simulink model "PendulumCart_Block"  (R2020a)
settings: Solver=ode45  StartTime=0.0  StopTime=12  RelTol=1e-3  EnableMultiTasking=on
values from neighbouring files (symbols this model uses):
  calGain = 1/dcgain(cltf)    [TP.m]
  g = 9.81    [TP.m]
  K = acker(A,B,phi)    [TP.m]
  l = 1    [TP.m]
  m = 0.5    [TP.m]
  M = 2    [TP.m]
  theta_0 = 0    [TP.m]
  theta_dot_0 = 0    [TP.m]
  x_0 = 0    [TP.m]
  x_dot_0 = 0    [TP.m]
settings Model: Creator=rodrigue  LastModifiedBy=m214134
settings DataIOCC: LimitDataPoints=on  SaveFormat=Array  ReturnWorkspaceOutputs=off
settings OptimizationCC: LifeSpan=inf
settings DebuggingCC: UnderspecifiedInitializationDetection=Classic  MergeDetectMultiDrivingBlocksExec=none  SolverPrmCheckMsg=warning  StateNameClashWarn=warning  SFUnexpectedBacktrackingDiag=warning  SFNoUnconditionalDefaultTransitionDiag=warning  SFExecutionAtInitializationDiag=none  ArithmeticOperatorsInVariantConditions=warning
settings HardwareCC: ProdBitPerPointer=32  ProdBitPerSizeT=32  ProdBitPerPtrDiffT=32  ProdLargestAtomicFloat=None  ProdIntDivRoundTo=Undefined  ProdEndianess=Unspecified  ProdWordSize=32  ProdHWDeviceType=32-bit Generic
settings ModelReferenceCC: PropagateSignalLabelsOutOfModel=off
settings SFSimCC: SimUseLocalCustomCode=off  CustomCodeUndefinedFunction=UseInterfaceOnly
settings RTWCC: RTWUseLocalCustomCode=off
settings CodeAppCC: StateflowObjectComments=on
settings GRTTargetCC: TargetLangStandard=C89/C90 (ANSI)
settings ConfigComp: CovMetricSettings=dw  CovHtmlReporting=on  CovSaveCumulativeToWorkspaceVar=on  CovSaveSingleToWorkspaceVar=on  CovExternalEMLEnable=off

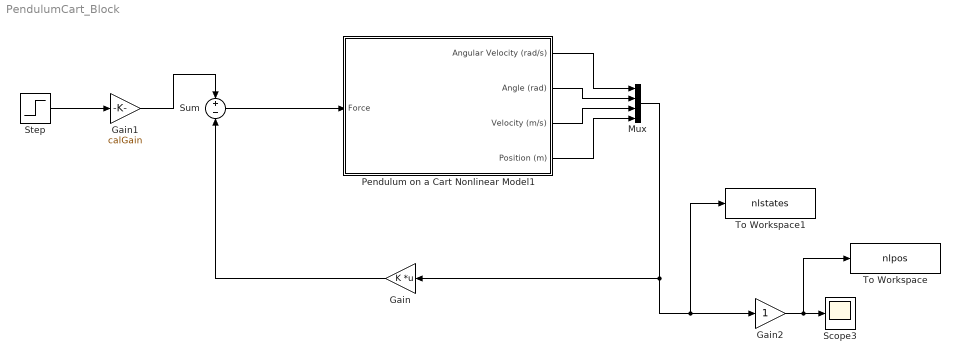
== system PendulumCart_Block ==
  Gain : Gain  Gain=K  Multiplication=Matrix(K*u)
  Gain1 : Gain  Gain=calGain
  Gain2 : Gain
  Mux : Mux
  Pendulum on a Cart Nonlinear Model1 : Subsystem  Description=Nonlinear of the Pendulum on a Cart. The input is the horizontal force applied to the cart.
      mask Display:
      | image('PendulumCartImage.jpg')
      | port_label('input', 1, 'F')
      | port_label('output', 1, 'Theta_dot')
      | port_label('output', 2, 'Theta')
      | port_label('output', 3, 'x_dot')
      | port_label('output', 4, 'x')
  Scope3 : Scope
  Step : Step  Time=0  SampleTime=0
  Sum : Sum  Inputs=+-
  To Workspace : ToWorkspace  VariableName=nlpos  SaveFormat=Timeseries  SampleTime=-1
  To Workspace1 : ToWorkspace  VariableName=nlstates  SaveFormat=Timeseries  SampleTime=-1
  wires:
  Pendulum on a Cart Nonlinear Model1/1(Angular Velocity (rad/s)) -> Mux/1
  Pendulum on a Cart Nonlinear Model1/2(Angle (rad)) -> Mux/2
  Pendulum on a Cart Nonlinear Model1/3(Velocity (m/s)) -> Mux/3
  Pendulum on a Cart Nonlinear Model1/4(Position (m)) -> Mux/4
  Mux/1 -> To Workspace1/1, Gain2/1, Gain/1
  Step/1 -> Gain1/1
  Gain1/1 -> Sum/1
  Gain/1 -> Sum/2
  Sum/1 -> Pendulum on a Cart Nonlinear Model1/1(Force)
  Gain2/1 -> To Workspace/1, Scope3/1

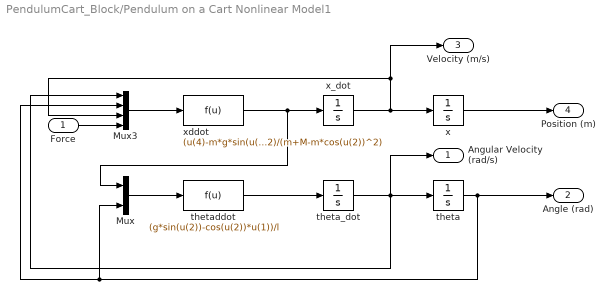
== system PendulumCart_Block/Pendulum on a Cart Nonlinear Model1 ==
  Force : Inport
  Mux : Mux  Inputs=2
  Mux3 : Mux
  theta : Integrator  InitialCondition=theta_0  ContinuousStateAttributes='theta'
  theta_dot : Integrator  InitialCondition=theta_dot_0  ContinuousStateAttributes='thetadot'
  thetaddot : Fcn  Expr=(g*sin(u(2))-cos(u(2))*u(1))/l
  x : Integrator  InitialCondition=x_0  ContinuousStateAttributes='x'
  x_dot : Integrator  InitialCondition=x_dot_0  ContinuousStateAttributes='xdot'
  xddot : Fcn  Expr=(u(4)-m*g*sin(u(2))*cos(u(2))+m*l*sin(u(2))*u(1)^2)/(m+M-m*cos(u(2))^2)
  Angular Velocity (rad/s) : Outport
  Angle (rad) : Outport  Port=2
  Velocity (m/s) : Outport  Port=3
  Position (m) : Outport  Port=4
  wires:
  Mux3/1 -> xddot/1
  theta_dot/1 -> Angular Velocity (rad/s)/1, theta/1, Mux3/1
  Force/1 -> Mux3/4
  x_dot/1 -> Velocity (m/s)/1, Mux3/3, x/1
  Mux/1 -> thetaddot/1
  xddot/1 -> Mux/1, x_dot/1
  thetaddot/1 -> theta_dot/1
  theta/1 -> Mux/2, Mux3/2, Angle (rad)/1
  x/1 -> Position (m)/1
